simulink library "resonance_lib"  (R2022a)
settings: Solver=VariableStepAuto  StartTime=0.0  StopTime=10.0  RelTol=1e-3
undefined symbols (not defined in the file): i, jsin
settings Model: Creator=tstef  LastModifiedBy=thomas

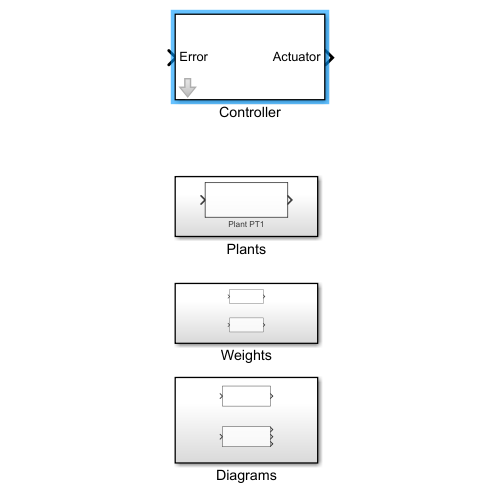
[thumbnail: Simulink's stored preview of the top-level diagram]
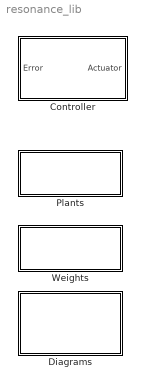
== system resonance_lib ==
  Controller : Subsystem  mask{k_P=0, k_I=0, k_R=95-390*i, k_Ra=950, k_Rb=-3.9e5, k_PIRA=9.3e5, k_PIRAp=-210, k_PIRAz=21, k_ILC=930, T1=0.094, T1p=-210, T1z=5, w0=100, zeta=0.05}
      mask prompts: k_P "Proportional Gain k_P (1):"; k_I "Integral Gain k_I (1):"; k_R "Resonant Gain k_R (complex):"; k_Ra "Resonant Gain k_Ra (1):"; k_Rb "Resonant Gain k_Rb (1):"; k_PIRA "PIRA Gain k_PIRA (1)::"; k_PIRAp "PIRA Pole (1):"; k_PIRAz "PIRA Zero (1):"; k_ILC "ILC Gain (1):"; T1 "Time Delay T1 (s):"; T1p "ILC Pole (s):"; T1z "ILC Zero (s):"; w0 "Resonant Frequency w0 (rad/s):"; zeta "Damping zeta (0-1):"
  Diagrams : Subsystem
  Plants : Subsystem
  Weights : Subsystem

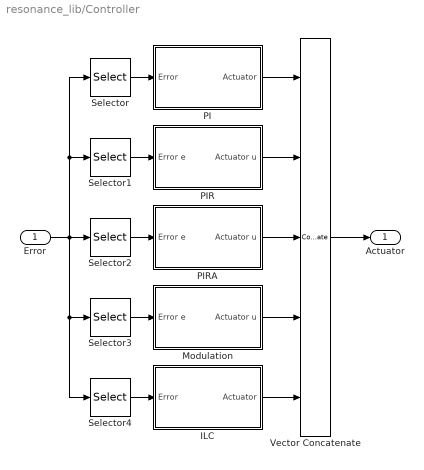
== system resonance_lib/Controller ==
  Error : Inport
  ILC : Subsystem  mask{k_P=0, k_I=k_I, k_R=k_ILC, w0=w0, zeta=zeta*2*exp(1), T1=T1, p=T1p, z=T1z}
      mask prompts: k_P "Proportional Gain k_P (1):"; k_I "Integral Gain k_I (1):"; k_R "Resonant Gain k_R (1):"; w0 "Resonant Frequency w0 (rad/s):"; zeta "Damping zeta (0-1):"; T1 "Part Delay (s):"; p "Filter Pole p (rad/s):"; z "Filter Zero z (rad/s):"
  Modulation : Subsystem  mask{k_P=k_P, k_I=k_I, k_R=k_R, w0=w0, zeta=zeta*w0}
      mask prompts: k_P "Proportional Gain k_P (1):"; k_I "Integral Gain k_I (1):"; k_R "Resonant Gain k_R (1):"; w0 "Resonant Frequency w0 (rad/s):"; zeta "Damping zeta (0-1):"
  PI : Subsystem  mask{k_P=k_P, k_I=k_I}
      mask prompts: k_P "Proportional Gain k_P (1):"; k_I "Integral Gain k_I (1):"
  PIR : Subsystem  mask{k_P=k_P, k_I=k_I, k_Ra=k_Ra, k_Rb=k_Rb, w0=w0, zeta=zeta}
      mask prompts: k_P "Proportional Gain k_P (1):"; k_I "Integral Gain k_I (1):"; k_Ra "Resonant Gain k_Ra (1):"; k_Rb "Resonant Gain k_Rb (1):"; w0 "Resonant Frequency w0 (rad/s):"; zeta "Damping zeta (0-1):"
  PIRA : Subsystem  mask{k_P=k_P, k_I=k_I, k_R=k_PIRA, p=k_PIRAp, z=k_PIRAz, w0=w0, zeta=zeta}
      mask prompts: k_P "Proportional Gain k_P (1):"; k_I "Integral Gain k_I (1):"; k_R "Resonant Gain k_R (1):"; p "PIRA Pole p (rad/s):"; z "PIRA Zero z (rad/s):"; w0 "Resonant Frequency w0 (rad/s):"; zeta "Damping zeta (0-1):"
  Selector : Selector  NumberOfDimensions=2  InputPortWidth=3  IndexOptions=Select all,Index vector (dialog)  Indices=1,1  OutputSizes=1,1
  Selector1 : Selector  NumberOfDimensions=2  InputPortWidth=3  IndexOptions=Select all,Index vector (dialog)  Indices=2,2  OutputSizes=1,1
  Selector2 : Selector  NumberOfDimensions=2  InputPortWidth=3  IndexOptions=Select all,Index vector (dialog)  Indices=3,3  OutputSizes=1,1
  Selector3 : Selector  NumberOfDimensions=2  InputPortWidth=3  IndexOptions=Select all,Index vector (dialog)  Indices=4,4  OutputSizes=1,1
  Selector4 : Selector  NumberOfDimensions=2  InputPortWidth=3  IndexOptions=Select all,Index vector (dialog)  Indices=5,5  OutputSizes=1,1
  Vector Concatenate : Concatenate  NumInputs=5  Mode=Multidimensional array  ConcatenateDimension=2
  Actuator : Outport
  wires:
  PI/1(Actuator) -> Vector Concatenate/1
  PIR/1(Actuator u) -> Vector Concatenate/2
  PIRA/1(Actuator u) -> Vector Concatenate/3
  Modulation/1(Actuator u) -> Vector Concatenate/4
  ILC/1(Actuator) -> Vector Concatenate/5
  Vector Concatenate/1 -> Actuator/1
  Selector1/1 -> PIR/1(Error e)
  Selector4/1 -> ILC/1(Error)
  Selector3/1 -> Modulation/1(Error e)
  Selector2/1 -> PIRA/1(Error e)
  Selector/1 -> PI/1(Error)
  Error/1 -> Selector4/1, Selector3/1, Selector/1, Selector1/1, Selector2/1

== system resonance_lib/Diagrams ==
  MS Design : Subsystem
  PI Design : Subsystem

== system resonance_lib/Plants ==
  Plant PT1 : Subsystem  mask{p=10}
      mask prompts: p "Pole p (rad/s):"

== system resonance_lib/Weights ==
  W_Int : Subsystem
  W_Res : Subsystem  mask{w=100, d=0.1}
      mask prompts: w "Resonance w (rad/s):"; d "Damping d (0-1):"

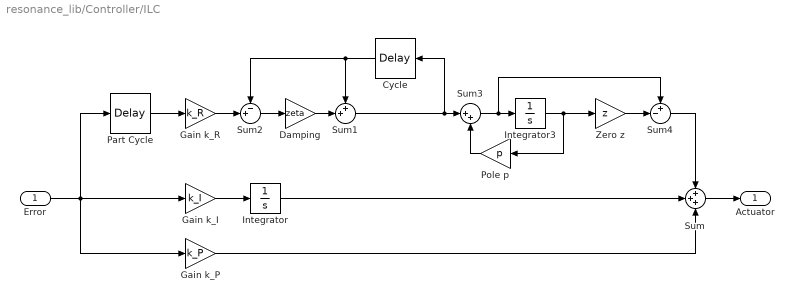
== system resonance_lib/Controller/ILC ==
  Error : Inport
  Cycle : TransportDelay  DelayTime=2*pi/w0  PadeOrder=20
  Damping : Gain  Gain=zeta
  Gain k_I : Gain  Gain=k_I
  Gain k_P : Gain  Gain=k_P
  Gain k_R : Gain  Gain=k_R
  Integrator : Integrator
  Integrator3 : Integrator
  Part Cycle : TransportDelay  DelayTime=T1  PadeOrder=20
  Pole p : Gain  Gain=p
  Sum : Sum  Inputs=+++
  Sum1 : Sum  Inputs=++|
  Sum2 : Sum  Inputs=-+|
  Sum3 : Sum  Inputs=|++
  Sum4 : Sum  Inputs=+-|
  Zero z : Gain  Gain=z
  Actuator : Outport
  wires:
  Damping/1 -> Sum1/2
  Gain k_R/1 -> Sum2/2
  Part Cycle/1 -> Gain k_R/1
  Cycle/1 -> Sum2/1, Sum1/1
  Sum1/1 -> Sum3/1, Cycle/1
  Sum2/1 -> Damping/1
  Error/1 -> Gain k_P/1, Gain k_I/1, Part Cycle/1
  Gain k_I/1 -> Integrator/1
  Sum/1 -> Actuator/1
  Integrator/1 -> Sum/2
  Zero z/1 -> Sum4/2
  Sum3/1 -> Sum4/1, Integrator3/1
  Integrator3/1 -> Zero z/1, Pole p/1
  Pole p/1 -> Sum3/2
  Sum4/1 -> Sum/1
  Gain k_P/1 -> Sum/3

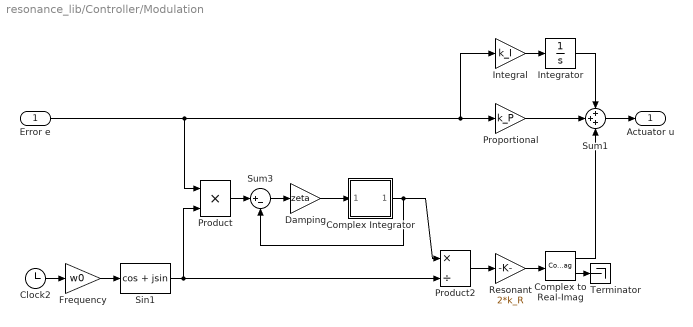
== system resonance_lib/Controller/Modulation ==
  Error e : Inport
  Clock2 : Clock
  Complex Integrator : Subsystem
  Complex to Real-Imag : ComplexToRealImag
  Damping : Gain  Gain=zeta
  Frequency : Gain  Gain=w0
  Integral : Gain  Gain=k_I
  Integrator : Integrator
  Product : Product
  Product2 : Product  Inputs=*/
  Proportional : Gain  Gain=k_P
  Resonant : Gain  Gain=2*k_R
  Sin1 : Trigonometry  Operator=cos + jsin
  Sum1 : Sum  Inputs=+++
  Sum3 : Sum  Inputs=|+-
  Terminator : Terminator
  Actuator u : Outport
  wires:
  Damping/1 -> Complex Integrator/1(In1)
  Complex Integrator/1(Out1) -> Sum3/2, Product2/1
  Sum3/1 -> Damping/1
  Resonant/1 -> Complex to Real-Imag/1
  Sum1/1 -> Actuator u/1
  Complex to Real-Imag/1 -> Sum1/3
  Complex to Real-Imag/2 -> Terminator/1
  Product2/1 -> Resonant/1
  Sin1/1 -> Product2/2, Product/2
  Product/1 -> Sum3/1
  Clock2/1 -> Frequency/1
  Frequency/1 -> Sin1/1
  Error e/1 -> Proportional/1, Integral/1, Product/1
  Integrator/1 -> Sum1/1
  Integral/1 -> Integrator/1
  Proportional/1 -> Sum1/2

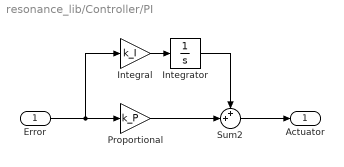
== system resonance_lib/Controller/PI ==
  Error : Inport
  Integral : Gain  Gain=k_I
  Integrator : Integrator
  Proportional : Gain  Gain=k_P
  Sum2 : Sum  Inputs=++|
  Actuator : Outport
  wires:
  Proportional/1 -> Sum2/2
  Error/1 -> Integral/1, Proportional/1
  Sum2/1 -> Actuator/1
  Integral/1 -> Integrator/1
  Integrator/1 -> Sum2/1

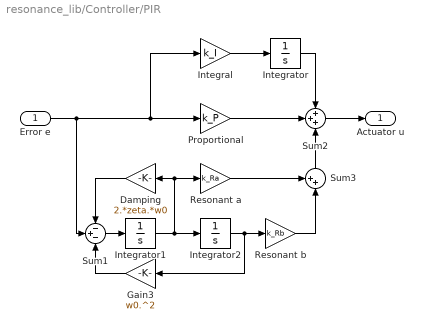
== system resonance_lib/Controller/PIR ==
  Error e : Inport
  Damping : Gain  Gain=2.*zeta.*w0
  Gain3 : Gain  Gain=w0.^2
  Integral : Gain  Gain=k_I
  Integrator : Integrator
  Integrator1 : Integrator
  Integrator2 : Integrator
  Proportional : Gain  Gain=k_P
  Resonant a : Gain  Gain=k_Ra
  Resonant b : Gain  Gain=k_Rb
  Sum1 : Sum  Inputs=-+-
  Sum2 : Sum  Inputs=+++
  Sum3 : Sum  Inputs=++|
  Actuator u : Outport
  wires:
  Integrator/1 -> Sum2/1
  Integral/1 -> Integrator/1
  Sum2/1 -> Actuator u/1
  Error e/1 -> Proportional/1, Integral/1, Sum1/2
  Proportional/1 -> Sum2/2
  Sum1/1 -> Integrator1/1
  Integrator1/1 -> Integrator2/1, Resonant a/1, Damping/1
  Integrator2/1 -> Resonant b/1, Gain3/1
  Resonant a/1 -> Sum3/1
  Damping/1 -> Sum1/1
  Resonant b/1 -> Sum3/2
  Sum3/1 -> Sum2/3
  Gain3/1 -> Sum1/3

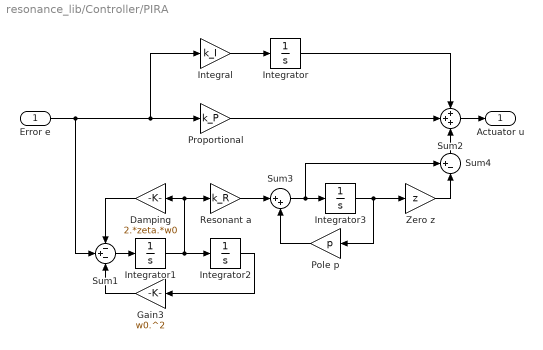
== system resonance_lib/Controller/PIRA ==
  Error e : Inport
  Damping : Gain  Gain=2.*zeta.*w0
  Gain3 : Gain  Gain=w0.^2
  Integral : Gain  Gain=k_I
  Integrator{,1..3} (4 alike) : Integrator
  Pole p : Gain  Gain=p
  Proportional : Gain  Gain=k_P
  Resonant a : Gain  Gain=k_R
  Sum1 : Sum  Inputs=-+-
  Sum2 : Sum  Inputs=+++
  Sum3 : Sum  Inputs=|++
  Sum4 : Sum  Inputs=+-|
  Zero z : Gain  Gain=z
  Actuator u : Outport
  wires:
  Integrator/1 -> Sum2/1
  Integral/1 -> Integrator/1
  Sum2/1 -> Actuator u/1
  Error e/1 -> Proportional/1, Integral/1, Sum1/2
  Proportional/1 -> Sum2/2
  Sum1/1 -> Integrator1/1
  Integrator1/1 -> Integrator2/1, Resonant a/1, Damping/1
  Integrator2/1 -> Gain3/1
  Damping/1 -> Sum1/1
  Gain3/1 -> Sum1/3
  Resonant a/1 -> Sum3/1
  Sum3/1 -> Sum4/1, Integrator3/1
  Zero z/1 -> Sum4/2
  Pole p/1 -> Sum3/2
  Integrator3/1 -> Zero z/1, Pole p/1
  Sum4/1 -> Sum2/3

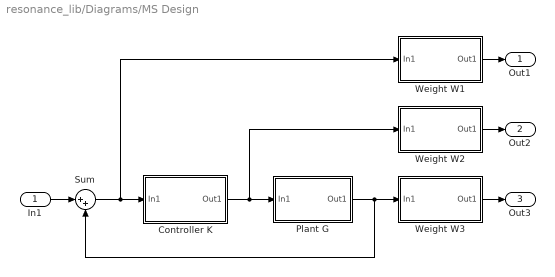
== system resonance_lib/Diagrams/MS Design ==
  In1 : Inport
  Controller K : Subsystem
  Plant G : Subsystem
  Sum : Sum  Inputs=|++
  Weight W1 : Subsystem
  Weight W2 : Subsystem
  Weight W3 : Subsystem
  Out1 : Outport
  Out2 : Outport  Port=2
  Out3 : Outport  Port=3
  wires:
  Controller K/1(Out1) -> Weight W2/1(In1), Plant G/1(In1)
  Sum/1 -> Weight W1/1(In1), Controller K/1(In1)
  In1/1 -> Sum/1
  Plant G/1(Out1) -> Weight W3/1(In1), Sum/2
  Weight W1/1(Out1) -> Out1/1
  Weight W2/1(Out1) -> Out2/1
  Weight W3/1(Out1) -> Out3/1

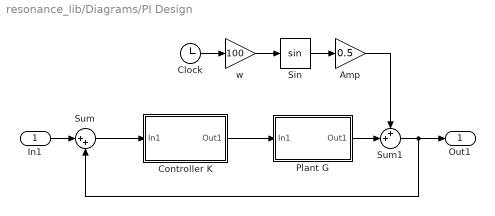
== system resonance_lib/Diagrams/PI Design ==
  In1 : Inport
  Amp : Gain  Gain=0.5
  Clock : Clock
  Controller K : Subsystem
  Plant G : Subsystem
  Sin : Trigonometry
  Sum : Sum  Inputs=|++
  Sum1 : Sum  Inputs=++|
  w : Gain  Gain=100
  Out1 : Outport
  wires:
  Sum1/1 -> Out1/1, Sum/2
  In1/1 -> Sum/1
  Sum/1 -> Controller K/1(In1)
  Controller K/1(Out1) -> Plant G/1(In1)
  Plant G/1(Out1) -> Sum1/2
  Sin/1 -> Amp/1
  w/1 -> Sin/1
  Clock/1 -> w/1
  Amp/1 -> Sum1/1

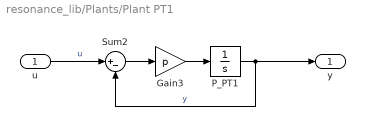
== system resonance_lib/Plants/Plant PT1 ==
  u : Inport
  Gain3 : Gain  Gain=p
  P_PT1 : Integrator
  Sum2 : Sum  Inputs=|+-
  y : Outport
  wires:
  u/1 -> Sum2/1  "u"
  Sum2/1 -> Gain3/1
  P_PT1/1 -> Sum2/2, y/1  "y"
  Gain3/1 -> P_PT1/1

== system resonance_lib/Weights/W_Int ==
  u : Inport
  W_Int : Integrator
  y : Outport
  wires:
  u/1 -> W_Int/1  "u"
  W_Int/1 -> y/1  "z"

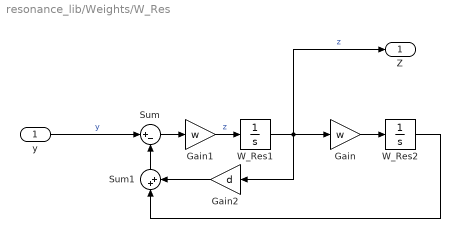
== system resonance_lib/Weights/W_Res ==
  y : Inport
  Gain : Gain  Gain=w
  Gain1 : Gain  Gain=w
  Gain2 : Gain  Gain=d
  Sum : Sum  Inputs=|+-
  Sum1 : Sum  Inputs=|++
  W_Res1 : Integrator
  W_Res2 : Integrator
  Z : Outport
  wires:
  Sum1/1 -> Sum/2
  y/1 -> Sum/1  "y"
  Sum/1 -> Gain1/1
  W_Res2/1 -> Sum1/1
  Gain2/1 -> Sum1/2
  W_Res1/1 -> Z/1, Gain2/1, Gain/1  "z"
  Gain1/1 -> W_Res1/1  "z"
  Gain/1 -> W_Res2/1

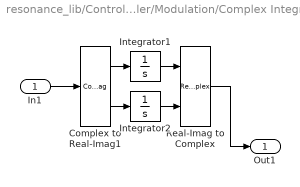
== system resonance_lib/Controller/Modulation/Complex Integrator ==
  In1 : Inport
  Complex to Real-Imag1 : ComplexToRealImag
  Integrator1 : Integrator
  Integrator2 : Integrator
  Real-Imag to Complex : RealImagToComplex
  Out1 : Outport
  wires:
  In1/1 -> Complex to Real-Imag1/1
  Integrator2/1 -> Real-Imag to Complex/2
  Complex to Real-Imag1/2 -> Integrator2/1
  Integrator1/1 -> Real-Imag to Complex/1
  Real-Imag to Complex/1 -> Out1/1
  Complex to Real-Imag1/1 -> Integrator1/1

== system resonance_lib/Diagrams/MS Design/Controller K ==
  In1 : Inport
  Out1 : Outport
  wires:
  In1/1 -> Out1/1

== system resonance_lib/Diagrams/MS Design/Plant G ==
  In1 : Inport
  Out1 : Outport
  wires:
  In1/1 -> Out1/1

== system resonance_lib/Diagrams/MS Design/Weight W1 ==
  In1 : Inport
  Out1 : Outport
  wires:
  In1/1 -> Out1/1

== system resonance_lib/Diagrams/MS Design/Weight W2 ==
  In1 : Inport
  Out1 : Outport
  wires:
  In1/1 -> Out1/1

== system resonance_lib/Diagrams/MS Design/Weight W3 ==
  In1 : Inport
  Out1 : Outport
  wires:
  In1/1 -> Out1/1

== system resonance_lib/Diagrams/PI Design/Controller K ==
  In1 : Inport
  Out1 : Outport
  wires:
  In1/1 -> Out1/1

== system resonance_lib/Diagrams/PI Design/Plant G ==
  In1 : Inport
  Out1 : Outport
  wires:
  In1/1 -> Out1/1
